simulink model "water_temp_change"  (R2024b)
settings: Solver=VariableStepAuto  StartTime=0.0  StopTime=inf  RelTol=1e-3
settings Model: Creator=KHALID  LastModifiedBy=KHALID

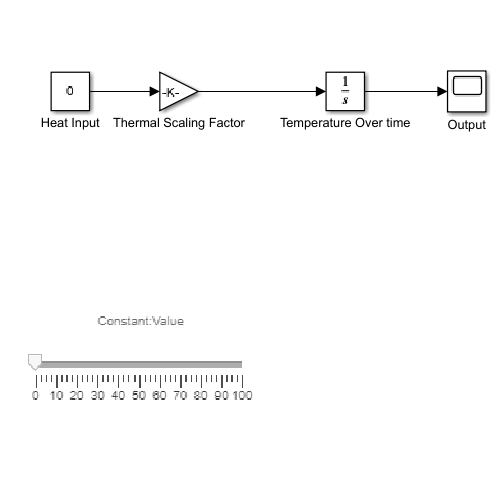
[thumbnail: Simulink's stored preview of the top-level diagram]
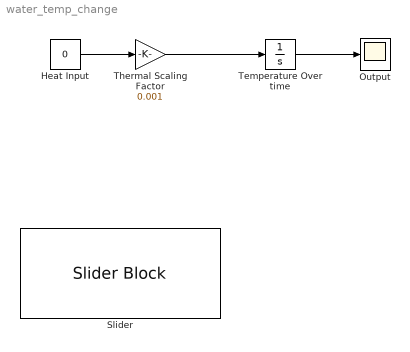
== system water_temp_change ==
  Heat Input : Constant  Value=0
  Output : Scope
  Slider : SliderBlock
  Temperature Over time : Integrator
  Thermal Scaling Factor : Gain  Gain=0.001
  wires:
  Thermal Scaling Factor/1 -> Temperature Over time/1
  Heat Input/1 -> Thermal Scaling Factor/1
  Temperature Over time/1 -> Output/1
